simulink model "sampleModel1504_1_sub"  (R2023a)
settings: Solver=VariableStepAuto  StartTime=0.0  StopTime=10.0  RelTol=1e-3
libraries: hdlsllib x6
settings Model: Creator=user1  LastModifiedBy=user1

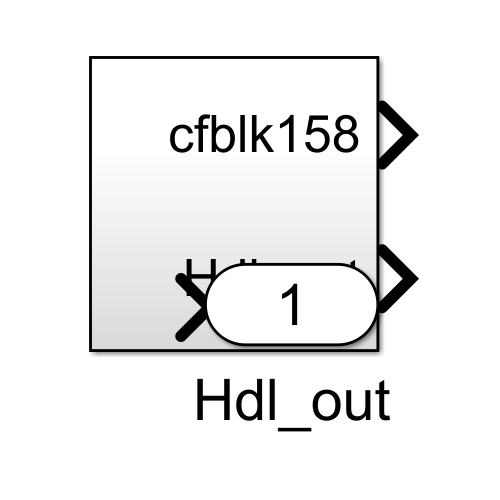
[thumbnail: Simulink's stored preview of the top-level diagram]
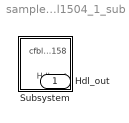
== system sampleModel1504_1_sub ==
  Subsystem : Subsystem
  Hdl_out : Outport  OutDataTypeStr=uint8

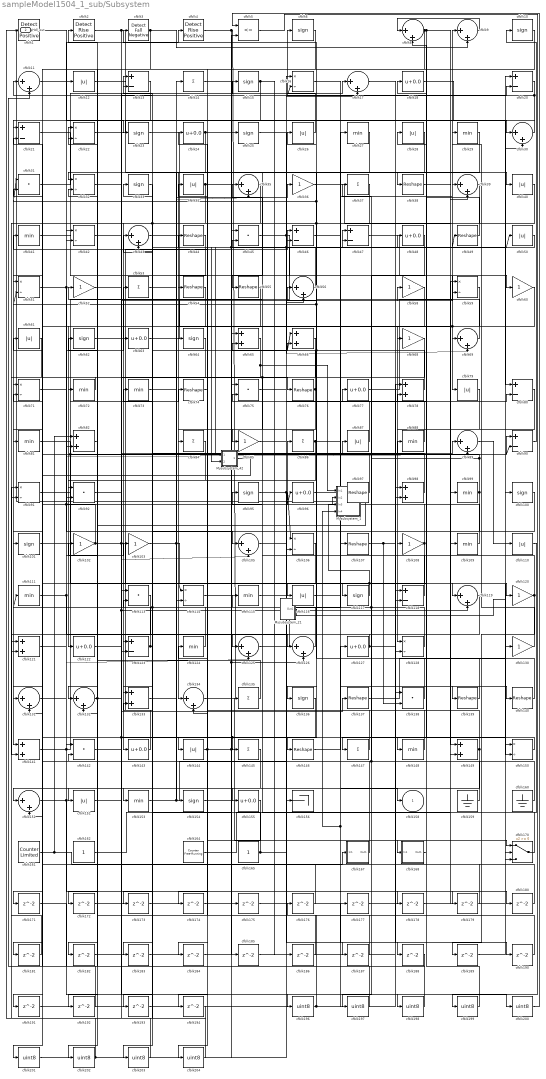
== system sampleModel1504_1_sub/Subsystem ==
  Mysubsystem_1 : Subsystem  TreatAsAtomicUnit=on  RTWFcnName=Mysubsystem_1
      settings: RTWFcnNameOpts=User specified  RTWFileNameOpts=Use function name
  Mysubsystem_21 : Subsystem  TreatAsAtomicUnit=on  RTWFcnName=Mysubsystem_21
      settings: RTWFcnNameOpts=User specified  RTWFileNameOpts=Use function name
  Mysubsystem_42 : Subsystem  TreatAsAtomicUnit=on  RTWFcnName=Mysubsystem_42
      settings: RTWFcnNameOpts=User specified  RTWFileNameOpts=Use function name
  cfblk1 : hdlsllib/Logic and Bit Operations/Detect Rise Positive  vinit=0  OutDataTypeStr=uint8
  cfblk{6,10,15,23,25,33,62,64,95,100..101,117,136,154} (14 alike) : Signum
  cfblk{36,52,58,60,68,85,102..103,108,120,130} (11 alike) : Gain  OutDataTypeStr=uint8
  cfblk{8..9,11,17,30,35,39,43,56,69,89,105,119,125..126,131..132,134,151} (19 alike) : Sum  Inputs=|++  OutDataTypeStr=uint8
  cfblk{16,22,32,42,51,59,71,91,106,114,128,150} (12 alike) : Product  Inputs=*/  OutDataTypeStr=uint8  RndMeth=Zero  SaturateOnIntegerOverflow=on
  cfblk{38,44,49,54..55,74,76,97,107,137,139..140,146} (13 alike) : Reshape
  cfblk{27,29,41,72..73,81,88,99,109,111,115,124,148,153} (14 alike) : MinMax  OutDataTypeStr=uint8
  cfblk{12,26,28,34,40,50,61,79,87,110,116,144,152} (13 alike) : Abs  OutDataTypeStr=uint8  SaturateOnIntegerOverflow=off
  cfblk{31,45,75,92,113,138,142} (7 alike) : DotProduct  OutDataTypeStr=uint8
  cfblk{13,20..21,46..47,80,90,118,123} (9 alike) : Sum  Inputs=+-  OutDataTypeStr=uint8
  cfblk{65..66,78,82,98,121,133,141,149} (9 alike) : Sum  OutDataTypeStr=uint8
  cfblk{18,24,48,63,77,96,122,127,143,155} (10 alike) : Bias  Bias=0.0  SaturateOnIntegerOverflow=off
  cfblk{14,37,53,84,86,135,145,147} (8 alike) : Sum  Inputs=+  OutDataTypeStr=uint8
  cfblk156 : Terminator
  cfblk159 : Ground
  cfblk160 : Ground
  cfblk161 : hdlsllib/Sources/Counter Limited  uplimit=7  tsamp=-1
  cfblk162 : Constant  OutDataTypeStr=uint8  SampleTime=-1
  cfblk164 : hdlsllib/Sources/Counter Free-Running  NumBits=16  tsamp=-1
  cfblk165 : Constant  OutDataTypeStr=uint8  SampleTime=-1
  cfblk167 : Subsystem
      settings: LibrarySourceBlock=|
      | hdlsllib/Ports &
      | Subsystems/Subsystem
  cfblk168 : Subsystem
      settings: LibrarySourceBlock=|
      | hdlsllib/Ports &
      | Subsystems/Subsystem
  cfblk170 : Switch  OutDataTypeStr=uint8  SaturateOnIntegerOverflow=off  InputSameDT=off
  cfblk{171..194} (24 alike) : Delay  SampleTime=1
  cfblk{196..204} (9 alike) : DataTypeConversion  OutDataTypeStr=uint8  SaturateOnIntegerOverflow=off  RndMeth=Floor
  cfblk2 : hdlsllib/Logic and Bit Operations/Detect Rise Positive  vinit=0  OutDataTypeStr=uint8
  cfblk3 : hdlsllib/Logic and Bit Operations/Detect Fall Negative  vinit=0  OutDataTypeStr=uint8
  cfblk4 : hdlsllib/Logic and Bit Operations/Detect Rise Positive  vinit=0  OutDataTypeStr=uint8
  cfblk5 : RelationalOperator  Operator=<=  OutDataTypeStr=boolean  InputSameDT=off
  cfblk158 : Outport  OutDataTypeStr=uint8  VectorParamsAs1DForOutWhenUnconnected=off
  Hdl_out : Outport  Port=2  OutDataTypeStr=uint8
  wires:
  cfblk15/1 -> cfblk186/1, cfblk141/1
  cfblk63/1 -> cfblk58/1
  cfblk8/1 -> cfblk152/1, cfblk39/2, cfblk117/1
  cfblk143/1 -> cfblk46/1
  cfblk123/1 -> cfblk102/1, cfblk153/1
  cfblk136/1 -> cfblk171/1, cfblk145/1
  cfblk81/1 -> cfblk90/2, cfblk120/1
  cfblk35/1 -> cfblk134/1
  cfblk144/1 -> cfblk124/1, cfblk168/1(In1), cfblk126/2, cfblk66/2
  cfblk140/1 -> cfblk97/1
  cfblk160/1 -> cfblk132/2, cfblk47/1
  cfblk27/1 -> cfblk64/1
  cfblk23/1 -> cfblk128/1
  cfblk30/1 -> cfblk21/1
  cfblk133/1 -> cfblk36/1
  cfblk79/1 -> cfblk108/1
  cfblk110/1 -> cfblk144/1
  cfblk3/1 -> cfblk9/2, cfblk101/1
  cfblk165/1 -> cfblk17/2, cfblk33/1
  cfblk107/1 -> cfblk138/2, cfblk140/1
  cfblk168/1(Out1) -> cfblk18/1
  cfblk134/1 -> cfblk170/1
  cfblk47/1 -> cfblk79/1
  cfblk89/1 -> cfblk110/1
  cfblk39/1 -> cfblk143/1
  cfblk167/1(Out1) -> cfblk61/1
  cfblk77/1 -> cfblk9/1
  cfblk152/1 -> cfblk137/1
  cfblk43/1 -> cfblk99/1
  cfblk4/1 -> cfblk126/1, cfblk135/1
  cfblk142/1 -> cfblk196/1
  cfblk148/1 -> cfblk41/1
  cfblk73/1 -> cfblk14/1
  cfblk64/1 -> cfblk131/1
  cfblk102/1 -> cfblk71/2, cfblk105/2, cfblk116/1
  cfblk117/1 -> cfblk114/1, Mysubsystem_1/3(In3)
  cfblk120/1 -> cfblk189/1, cfblk52/1
  cfblk34/1 -> cfblk38/1, cfblk173/1, cfblk91/2
  cfblk141/1 -> cfblk63/1, cfblk48/1
  cfblk95/1 -> cfblk187/1, cfblk106/1
  cfblk9/1 -> cfblk8/1
  cfblk42/1 -> cfblk179/1, cfblk150/2
  cfblk17/1 -> cfblk60/1
  cfblk55/1 -> cfblk122/1
  cfblk147/1 -> cfblk115/1
  cfblk38/1 -> cfblk109/1
  cfblk26/1 -> cfblk6/1
  cfblk109/1 -> cfblk86/1
  cfblk164/1 -> cfblk59/1
  cfblk91/1 -> cfblk74/1
  cfblk114/1 -> cfblk50/1, Mysubsystem_42/1(In1)
  cfblk161/1 -> cfblk82/1, cfblk167/1(In1)
  cfblk149/1 -> cfblk201/1, cfblk47/2
  cfblk74/1 -> cfblk24/1
  cfblk153/1 -> cfblk90/1, cfblk106/2
  cfblk36/1 -> cfblk149/1
  cfblk103/1 -> cfblk35/2, cfblk130/1
  cfblk127/1 -> cfblk190/1, cfblk123/1
  cfblk85/1 -> cfblk77/1
  cfblk99/1 -> cfblk133/1, cfblk37/1, cfblk31/2
  cfblk21/1 -> cfblk98/2
  cfblk2/1 -> cfblk198/1, cfblk154/1
  cfblk115/1 -> cfblk88/1
  cfblk12/1 -> cfblk107/1
  cfblk22/1 -> cfblk30/1
  cfblk51/1 -> cfblk105/1, cfblk12/1
  cfblk87/1 -> cfblk45/2
  cfblk118/1 -> cfblk56/1
  cfblk29/1 -> cfblk55/1
  cfblk137/1 -> cfblk100/1
  cfblk116/1 -> cfblk158/1
  cfblk44/1 -> cfblk54/1
  cfblk31/1 -> cfblk15/1
  cfblk86/1 -> cfblk39/1, cfblk92/1
  cfblk82/1 -> cfblk2/1
  cfblk151/1 -> cfblk178/1, cfblk125/2
  cfblk122/1 -> cfblk59/2
  cfblk145/1 -> cfblk155/1
  cfblk162/1 -> cfblk25/1
  cfblk78/1 -> cfblk13/1
  cfblk62/1 -> cfblk53/1
  cfblk32/1 -> cfblk76/1
  cfblk146/1 -> cfblk127/1
  cfblk119/1 -> cfblk141/2
  cfblk69/1 -> cfblk31/1, cfblk3/1
  cfblk130/1 -> cfblk29/1
  cfblk90/1 -> cfblk10/1
  cfblk45/1 -> cfblk69/2, cfblk118/1
  cfblk50/1 -> cfblk46/2
  cfblk108/1 -> cfblk192/1, Mysubsystem_1/2(In2)
  cfblk125/1 -> cfblk27/1
  cfblk28/1 -> cfblk136/1
  cfblk72/1 -> cfblk71/1
  cfblk24/1 -> cfblk40/1, cfblk32/1
  cfblk40/1 -> cfblk146/1, cfblk81/1
  cfblk18/1 -> cfblk80/1
  cfblk159/1 -> cfblk35/1
  cfblk97/1 -> cfblk34/1
  cfblk66/1 -> cfblk85/1, cfblk92/2
  cfblk49/1 -> cfblk8/2
  cfblk20/1 -> cfblk16/2, cfblk84/1
  cfblk101/1 -> cfblk156/1
  cfblk132/1 -> cfblk32/2, cfblk119/2, cfblk89/1
  cfblk11/1 -> cfblk4/1
  cfblk113/1 -> cfblk202/1
  cfblk150/1 -> cfblk147/1
  cfblk10/1 -> cfblk72/1
  cfblk170/1 -> cfblk78/2
  cfblk56/1 -> cfblk11/1
  cfblk88/1 -> cfblk75/2
  cfblk13/1 -> cfblk51/1
  cfblk135/1 -> cfblk22/1
  cfblk52/1 -> cfblk20/2
  cfblk76/1 -> cfblk174/1, cfblk65/2
  cfblk126/1 -> cfblk95/1
  cfblk121/1 -> cfblk103/1
  cfblk124/1 -> cfblk73/1, cfblk62/1
  cfblk128/1 -> cfblk111/1, cfblk87/1
  cfblk131/1 -> cfblk42/1
  cfblk105/1 -> cfblk119/1
  cfblk61/1 -> cfblk121/2
  cfblk139/1 -> cfblk66/1, cfblk51/2, cfblk26/1
  cfblk98/1 -> cfblk43/2
  cfblk1/1 -> cfblk23/1
  cfblk100/1 -> cfblk114/2
  cfblk65/1 -> cfblk82/2, Mysubsystem_1/1(In1)
  cfblk41/1 -> cfblk123/2
  cfblk106/1 -> cfblk151/1
  cfblk16/1 -> Mysubsystem_1/4(In4), cfblk188/1
  cfblk60/1 -> cfblk151/2, cfblk69/1
  cfblk25/1 -> cfblk56/2
  cfblk84/1 -> cfblk132/1
  cfblk80/1 -> cfblk148/1
  cfblk96/1 -> cfblk80/2, cfblk139/1
  cfblk111/1 -> cfblk125/1, cfblk89/2, cfblk96/1
  cfblk138/1 -> cfblk44/1
  cfblk71/1 -> cfblk42/2
  cfblk92/1 -> cfblk17/1
  cfblk53/1 -> cfblk68/1
  cfblk75/1 -> cfblk49/1, Mysubsystem_42/2(In2)
  cfblk59/1 -> cfblk172/1
  cfblk172/1 -> cfblk98/1
  cfblk173/1 -> cfblk45/1
  cfblk174/1 -> cfblk170/2
  cfblk154/1 -> cfblk175/1
  cfblk175/1 -> cfblk149/2
  cfblk176/1 -> cfblk65/1
  cfblk177/1 -> cfblk30/2
  cfblk178/1 -> cfblk20/1
  cfblk179/1 -> cfblk131/2
  cfblk46/1 -> cfblk180/1
  cfblk180/1 -> cfblk75/1
  cfblk181/1 -> cfblk91/1
  cfblk182/1 -> cfblk118/2
  cfblk58/1 -> cfblk183/1
  cfblk183/1 -> cfblk13/2
  cfblk68/1 -> cfblk184/1
  cfblk184/1 -> cfblk128/2
  cfblk14/1 -> cfblk185/1
  cfblk185/1 -> cfblk78/1
  cfblk186/1 -> cfblk133/2
  cfblk187/1 -> cfblk134/2
  cfblk188/1 -> cfblk11/2
  cfblk189/1 -> cfblk170/3
  cfblk190/1 -> cfblk22/2
  cfblk54/1 -> cfblk191/1
  cfblk191/1 -> cfblk138/1
  cfblk192/1 -> cfblk21/2
  cfblk37/1 -> cfblk193/1
  cfblk193/1 -> cfblk43/1
  cfblk6/1 -> cfblk194/1
  cfblk194/1 -> cfblk1/1
  cfblk196/1 -> cfblk176/1, cfblk177/1
  cfblk48/1 -> cfblk197/1
  cfblk197/1 -> cfblk142/1
  cfblk198/1 -> cfblk142/2
  cfblk5/1 -> cfblk199/1
  cfblk199/1 -> cfblk28/1
  cfblk171/1 -> cfblk200/1
  cfblk200/1 -> cfblk5/1
  cfblk201/1 -> cfblk5/2
  cfblk202/1 -> cfblk121/1, cfblk16/1
  cfblk33/1 -> cfblk203/1
  cfblk203/1 -> cfblk113/1
  cfblk155/1 -> cfblk204/1
  cfblk204/1 -> cfblk113/2
  Mysubsystem_1/1(Out1) -> Hdl_out/1, cfblk182/1
  Mysubsystem_21/1(Out1) -> cfblk150/1
  Mysubsystem_42/1(Out1) -> cfblk181/1

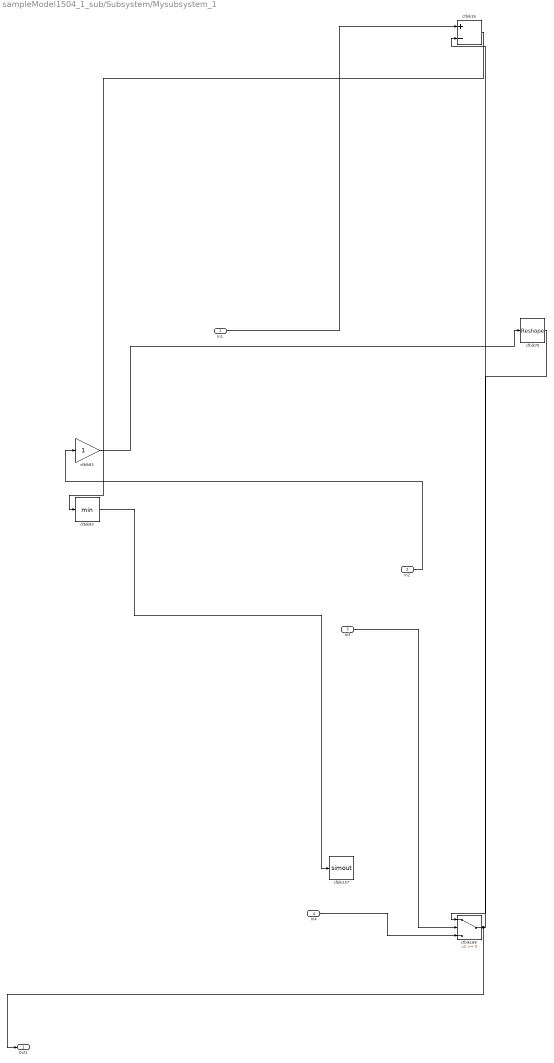
== system sampleModel1504_1_sub/Subsystem/Mysubsystem_1 ==
  In1 : Inport
  In2 : Inport  Port=2
  In3 : Inport  Port=3
  In4 : Inport  Port=4
  cfblk157 : ToWorkspace  VariableName=simout  SaveFormat=Timeseries  SampleTime=-1
  cfblk169 : Switch  SaturateOnIntegerOverflow=off  InputSameDT=off
  cfblk19 : Sum  Inputs=+-
  cfblk70 : Reshape
  cfblk83 : Gain
  cfblk93 : MinMax
  Out1 : Outport
  wires:
  In3/1 -> cfblk169/2
  In4/1 -> cfblk169/3
  cfblk70/1 -> cfblk169/1
  In1/1 -> cfblk19/1
  cfblk93/1 -> cfblk157/1
  In2/1 -> cfblk83/1
  cfblk83/1 -> cfblk70/1
  cfblk169/1 -> cfblk19/2, Out1/1
  cfblk19/1 -> cfblk93/1

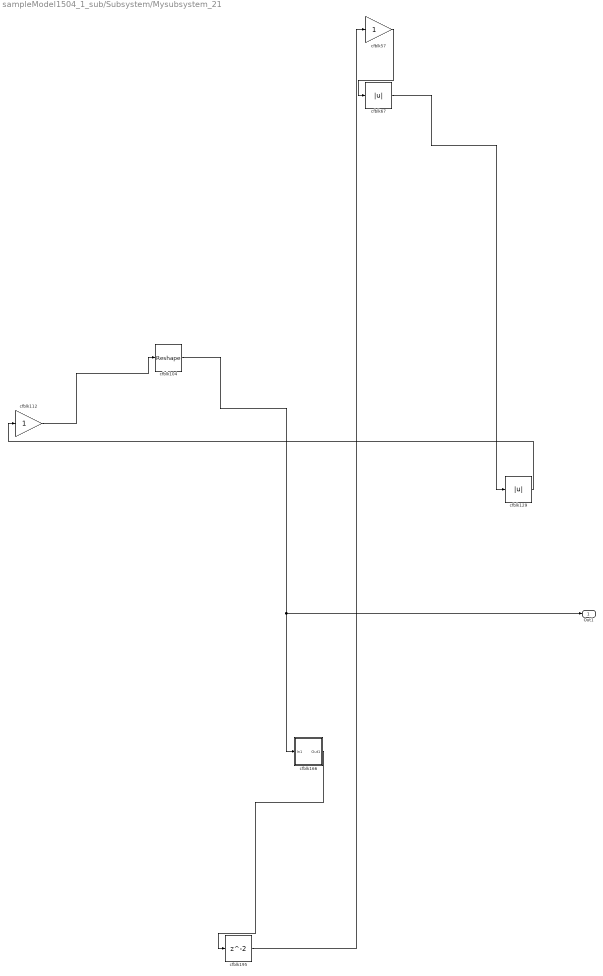
== system sampleModel1504_1_sub/Subsystem/Mysubsystem_21 ==
  cfblk104 : Reshape
  cfblk112 : Gain
  cfblk129 : Abs  SaturateOnIntegerOverflow=off
  cfblk166 : Subsystem
      settings: LibrarySourceBlock=|
      | hdlsllib/Ports &
      | Subsystems/Subsystem
  cfblk195 : Delay  SampleTime=1
  cfblk57 : Gain
  cfblk67 : Abs  SaturateOnIntegerOverflow=off
  Out1 : Outport
  wires:
  cfblk57/1 -> cfblk67/1
  cfblk112/1 -> cfblk104/1
  cfblk129/1 -> cfblk112/1
  cfblk67/1 -> cfblk129/1
  cfblk195/1 -> cfblk57/1
  cfblk104/1 -> cfblk166/1(In1), Out1/1
  cfblk166/1(Out1) -> cfblk195/1

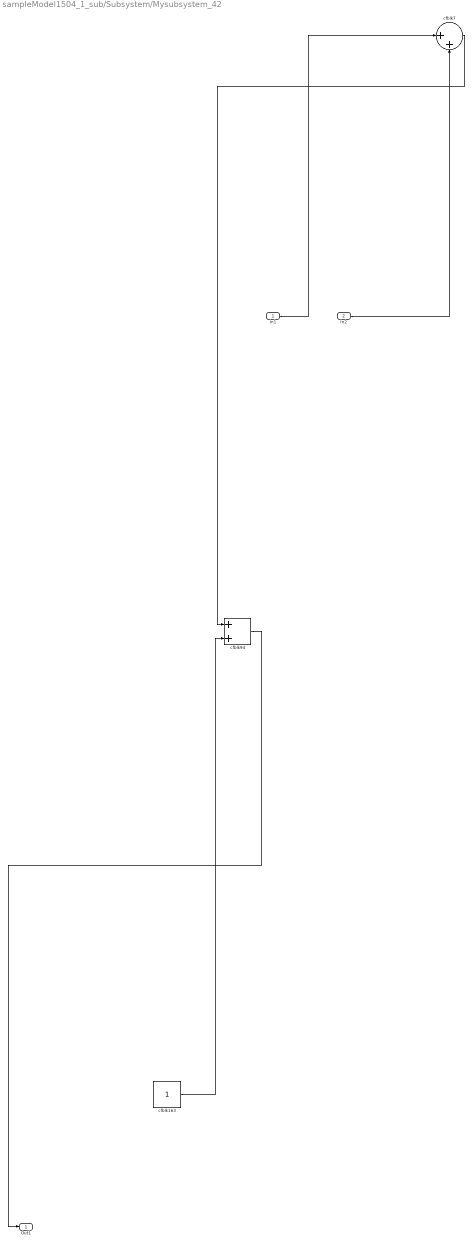
== system sampleModel1504_1_sub/Subsystem/Mysubsystem_42 ==
  In1 : Inport
  In2 : Inport  Port=2
  cfblk163 : Constant  SampleTime=-1
  cfblk7 : Sum  Inputs=|++
  cfblk94 : Sum
  Out1 : Outport
  wires:
  cfblk94/1 -> Out1/1
  In2/1 -> cfblk7/2
  cfblk163/1 -> cfblk94/2
  cfblk7/1 -> cfblk94/1
  In1/1 -> cfblk7/1

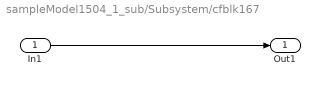
== system sampleModel1504_1_sub/Subsystem/cfblk167 ==
  In1 : Inport
  Out1 : Outport
  wires:
  In1/1 -> Out1/1

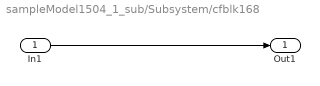
== system sampleModel1504_1_sub/Subsystem/cfblk168 ==
  In1 : Inport
  Out1 : Outport
  wires:
  In1/1 -> Out1/1

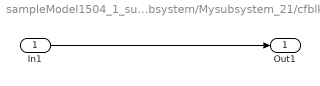
== system sampleModel1504_1_sub/Subsystem/Mysubsystem_21/cfblk166 ==
  In1 : Inport
  Out1 : Outport
  wires:
  In1/1 -> Out1/1
